simulink model "OpenLoop_Test"  (R2024a)
settings: Solver=VariableStepAuto  StartTime=0.0  StopTime=10.0  RelTol=1e-3
libraries: RCTblocks x6
settings Model: Creator=Thoma  LastModifiedBy=Thoma

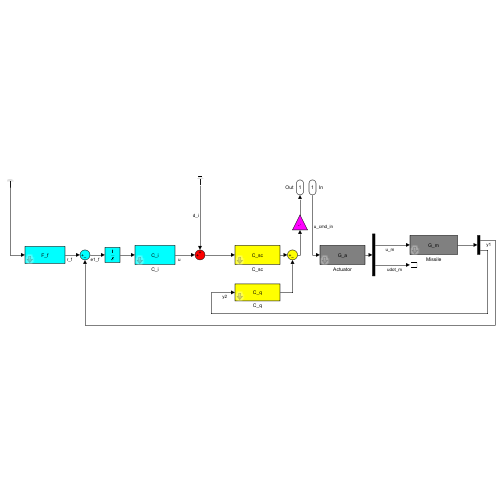
[thumbnail: Simulink's stored preview of the top-level diagram]
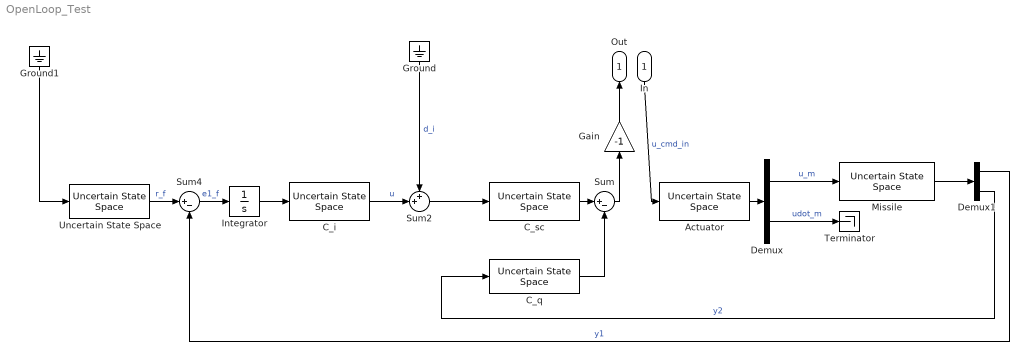
== system OpenLoop_Test ==
  In : Inport
  Actuator : RCTblocks/Uncertain State Space  Tag=USS  USystem=G_a  UValue=[]  X0=[]  uX0=[]
  C_i : RCTblocks/Uncertain State Space  Tag=USS  USystem=C_i  UValue=[]  X0=[]  uX0=[]
  C_q : RCTblocks/Uncertain State Space  Tag=USS  USystem=C_q  UValue=[]  X0=[]  uX0=[]
  C_sc : RCTblocks/Uncertain State Space  Tag=USS  USystem=C_sc  UValue=[]  X0=[]  uX0=[]
  Demux : Demux  Outputs=2
  Demux1 : Demux  Outputs=2
  Gain : Gain  Gain=-1
  Ground : Ground
  Ground1 : Ground
  Integrator : Integrator
  Missile : RCTblocks/Uncertain State Space  Tag=USS  USystem=G_m  UValue=[]  X0=[]  uX0=[]
  Sum : Sum  Inputs=|+-
  Sum2 : Sum  Inputs=++|
  Sum4 : Sum  Inputs=|+-
  Terminator : Terminator
  Uncertain State Space : RCTblocks/Uncertain State Space  Tag=USS  USystem=F_f  UValue=[]  X0=[]  uX0=[]
  Out : Outport
  wires:
  Demux1/1 -> Sum4/2  "y1"
  Actuator/1 -> Demux/1
  C_sc/1 -> Sum/1
  C_i/1 -> Sum2/2  "u"
  Demux/2 -> Terminator/1  "udot_m"
  Uncertain State Space/1 -> Sum4/1  "r_f"
  Sum2/1 -> C_sc/1
  Integrator/1 -> C_i/1
  Demux1/2 -> C_q/1  "y2"
  Demux/1 -> Missile/1  "u_m"
  C_q/1 -> Sum/2
  Sum/1 -> Gain/1
  Sum4/1 -> Integrator/1  "e1_f"
  Missile/1 -> Demux1/1
  Ground/1 -> Sum2/1  "d_i"
  Ground1/1 -> Uncertain State Space/1
  In/1 -> Actuator/1  "u_cmd_in"
  Gain/1 -> Out/1
